simulink model "et_robocon_dev_guy_arch_pi"  (R2013b)
settings: Solver=FixedStepDiscrete  SolverMode=SingleTasking  StartTime=0.0  StopTime=inf  FixedStep=balancer_ts  RelTol=1e-3
undefined symbols (not defined in the file): a_d, a_r, balancerStates_Bus0, Batt, battery_gain, battery_offset, cmd_max, current_mode_status, current_task_operation_status, DiscIntNeverNeededParam, exec_period, Init_Bus0, K, k_f, k_i, k_phidot, k_thetadot, lightCalib, R, STATE, TRACK_MODE_LIST, ts2, W
libraries: legonxtlib x28, simulink x19, simulink_extras x4
(part 3 of 4)

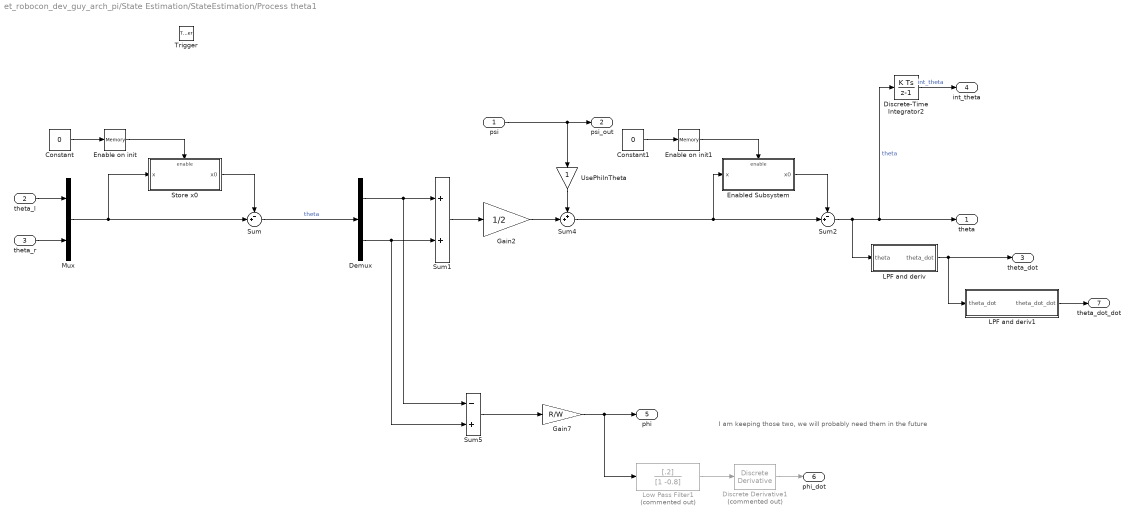
== system et_robocon_dev_guy_arch_pi/State Estimation/StateEstimation/Process theta1 ==
  note: I am keeping those two, we will probably need them in the future
  psi : Inport
  theta_l : Inport  Port=2
  theta_r : Inport  Port=3
  Trigger : TriggerPort  TriggerType=function-call  StatesWhenEnabling=reset  PortDimensions=1
  Constant : Constant  Value=0  OutDataTypeStr=boolean
  Constant1 : Constant  Value=0  OutDataTypeStr=boolean
  Demux : Demux  Outputs=2
  Discrete Derivative1 : simulink/Discrete/Discrete Derivative  Commented=on  gainval=1.0  ICPrevScaledInput=0.0  InputProcessing=Inherited  OutMin=[]  OutMax=[]  OutDataType=fixdt(1, 16)  OutScaling=2^-10  DoSatur=off
  Discrete-Time Integrator2 : DiscreteIntegrator  SampleTime=-1  ICPrevOutput=DiscIntNeverNeededParam  ICPrevScaledInput=DiscIntNeverNeededParam
  Enable on init : Memory  X0=1  InheritSampleTime=on
  Enable on init1 : Memory  X0=1  InheritSampleTime=on
  Enabled Subsystem : Subsystem  TreatAsAtomicUnit=on
  Gain2 : Gain  Gain=1/2
  Gain7 : Gain  Gain=R/W
  LPF and deriv : Subsystem
  LPF and deriv1 : Subsystem
  Low Pass Filter1 : DiscreteFilter  Commented=on  Numerator=[.2]  Denominator=[1 -0.8]
  Mux : Mux  Inputs=2
  Store x0 : Subsystem  TreatAsAtomicUnit=on
  Sum : Sum  Inputs=-+|
  Sum1 : Sum
  Sum2 : Sum  Inputs=-+|
  Sum4 : Sum  Inputs=++|
  Sum5 : Sum  Inputs=-+
  UsePhiInTheta : Gain
  theta : Outport  InitialOutput=0
  psi_out : Outport  Port=2  InitialOutput=0
  theta_dot : Outport  Port=3  OutputWhenDisabled=reset  InitialOutput=0
  int_theta : Outport  Port=4  InitialOutput=0
  phi : Outport  Port=5  OutputWhenDisabled=reset  InitialOutput=0
  phi_dot : Outport  Port=6  OutputWhenDisabled=reset  InitialOutput=0
  theta_dot_dot : Outport  Port=7  OutputWhenDisabled=reset  InitialOutput=0
  wires:
  Gain7/1 -> Low Pass Filter1/1, phi/1
  Sum5/1 -> Gain7/1
  Sum2/1 -> LPF and deriv/1(theta), theta/1, Discrete-Time Integrator2/1  "theta"
  Enabled Subsystem/1(x0) -> Sum2/1
  Constant1/1 -> Enable on init1/1
  Enable on init1/1 -> Enabled Subsystem/Enable
  Sum4/1 -> Sum2/2, Enabled Subsystem/1(x)
  Discrete-Time Integrator2/1 -> int_theta/1  "int_theta"
  psi/1 -> UsePhiInTheta/1, psi_out/1
  UsePhiInTheta/1 -> Sum4/1
  Sum1/1 -> Gain2/1
  Gain2/1 -> Sum4/2
  Demux/2 -> Sum1/2, Sum5/2
  Demux/1 -> Sum1/1, Sum5/1
  theta_r/1 -> Mux/2
  theta_l/1 -> Mux/1
  Mux/1 -> Sum/2, Store x0/1(x)
  Sum/1 -> Demux/1  "theta"
  Store x0/1(x0) -> Sum/1
  Constant/1 -> Enable on init/1
  Enable on init/1 -> Store x0/Enable
  Low Pass Filter1/1 -> Discrete Derivative1/1
  Discrete Derivative1/1 -> phi_dot/1
  LPF and deriv/1(theta_dot) -> LPF and deriv1/1(theta_dot), theta_dot/1
  LPF and deriv1/1(theta_dot_dot) -> theta_dot_dot/1

== system et_robocon_dev_guy_arch_pi/Main Controller/normal_operation_modes.line_tracking_after_seesaw/line_tracking_mode.Track.analyzeEncoders/AngleCounter/AngleCount_and_EncoderReset ==
  In1 : Inport
  In2 : Inport  Port=2  OutDataTypeStr=uint8
  Trigger : TriggerPort
  Data Store Read : DataStoreRead  Commented=on  DataStoreName=fwd_premode_last
  Data Store Write : DataStoreWrite  Commented=on  DataStoreName=fwd_postmode_init
  EC : Outport
  Cnt : Outport  Port=2  InitialOutput=1
  wires:
  In2/1 -> Cnt/1
  In1/1 -> EC/1
  Data Store Read/1 -> Data Store Write/1

== system et_robocon_dev_guy_arch_pi/Main Controller/normal_operation_modes.line_tracking_after_seesaw/line_tracking_mode.Track.analyzeEncoders/AngleCounter/Compute Distance ==
  R : Inport
  L : Inport  Port=2
  Gain1 : Gain  Gain=1/2
  Subtract : Sum
  EncoderMean : Outport
  wires:
  Gain1/1 -> EncoderMean/1
  Subtract/1 -> Gain1/1
  L/1 -> Subtract/2
  R/1 -> Subtract/1

== system et_robocon_dev_guy_arch_pi/Main Controller/normal_operation_modes.line_tracking_after_seesaw/line_tracking_mode.Track.analyzeEncoders/AngleCounter/Direction ==
  note: 160: Distance between left tire and right tire
      | 41: Radius of tire
  R : Inport
  L : Inport  Port=2
  Gain2 : Gain  Gain=41/160
  Subtract1 : Sum  Inputs=+-
  Angle : Outport
  wires:
  Gain2/1 -> Angle/1
  R/1 -> Subtract1/1
  L/1 -> Subtract1/2
  Subtract1/1 -> Gain2/1

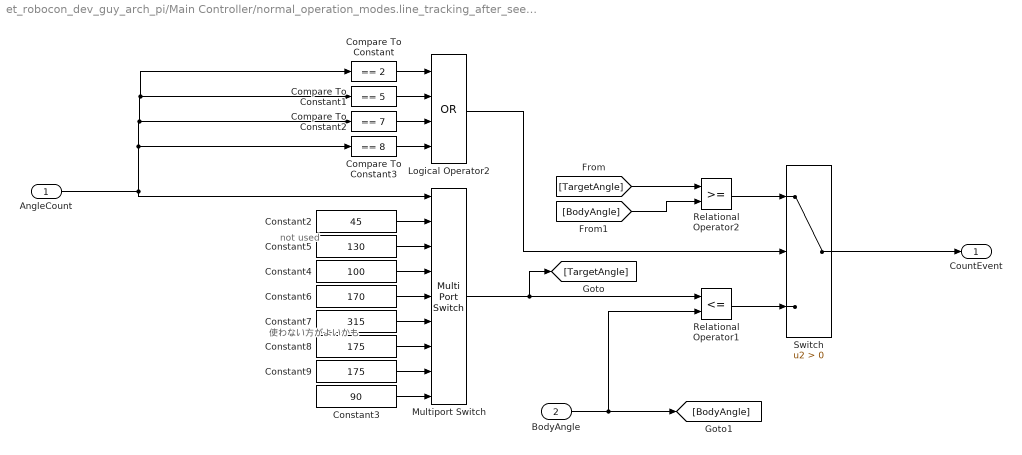
== system et_robocon_dev_guy_arch_pi/Main Controller/normal_operation_modes.line_tracking_after_seesaw/line_tracking_mode.Track.analyzeEncoders/AngleCounter/JudgeByAngle ==
  note: not used
  note: 使わない方がよいかも
  AngleCount : Inport
  BodyAngle : Inport  Port=2
  Compare To Constant : simulink/Logic and Bit Operations/Compare To Constant  relop===  const=2  OutDataTypeStr=boolean
  Compare To Constant1 : simulink/Logic and Bit Operations/Compare To Constant  relop===  const=5  OutDataTypeStr=boolean
  Compare To Constant2 : simulink/Logic and Bit Operations/Compare To Constant  relop===  const=7  OutDataTypeStr=boolean
  Compare To Constant3 : simulink/Logic and Bit Operations/Compare To Constant  relop===  const=8  OutDataTypeStr=boolean
  Constant2 : Constant  Value=45  OutDataTypeStr=int32
  Constant3 : Constant  Value=90  OutDataTypeStr=int32
  Constant4 : Constant  Value=100  OutDataTypeStr=int32
  Constant5 : Constant  Value=130  OutDataTypeStr=int32
  Constant6 : Constant  Value=170  OutDataTypeStr=int32
  Constant7 : Constant  Value=315  OutDataTypeStr=int32
  Constant8 : Constant  Value=175  OutDataTypeStr=int32
  Constant9 : Constant  Value=175  OutDataTypeStr=int32
  Logical Operator2 : Logic  Operator=OR  Inputs=4  AllPortsSameDT=off  OutDataTypeStr=boolean
  Multiport Switch : MultiPortSwitch  Inputs=8  DiagnosticForDefault=None
  Relational Operator1 : RelationalOperator  Operator=<=  OutDataTypeStr=boolean
  Relational Operator2 : RelationalOperator  OutDataTypeStr=boolean
  Switch : Switch  Criteria=u2 > Threshold
  CountEvent : Outport
  wires:
  Constant3/1 -> Multiport Switch/9
  Relational Operator1/1 -> Switch/3
  Compare To Constant2/1 -> Logical Operator2/3
  Compare To Constant3/1 -> Logical Operator2/4
  Compare To Constant1/1 -> Logical Operator2/2
  Compare To Constant/1 -> Logical Operator2/1
  Relational Operator2/1 -> Switch/1
  Logical Operator2/1 -> Switch/2
  AngleCount/1 -> Compare To Constant/1, Compare To Constant1/1, Compare To Constant2/1, Compare To Constant3/1, Multiport Switch/1
  BodyAngle/1 -> [BodyAngle], Relational Operator1/2
  Constant9/1 -> Multiport Switch/8
  Multiport Switch/1 -> [TargetAngle], Relational Operator1/1
  Constant4/1 -> Multiport Switch/4
  Constant8/1 -> Multiport Switch/7
  Constant5/1 -> Multiport Switch/3
  Constant2/1 -> Multiport Switch/2
  Constant6/1 -> Multiport Switch/5
  Constant7/1 -> Multiport Switch/6
  [BodyAngle] -> Relational Operator2/2
  [TargetAngle] -> Relational Operator2/1
  Switch/1 -> CountEvent/1

== system et_robocon_dev_guy_arch_pi/Main Controller/normal_operation_modes.line_tracking_after_seesaw/line_tracking_mode.Track.analyzeEncoders/AngleCounter/JudgeByDistance ==
  AngleCount : Inport
  Distance : Inport  Port=2
  Constant1 : Constant  Value=14700  OutDataTypeStr=int32
  Constant10 : Constant  Value=9700  OutDataTypeStr=int32
  Constant2 : Constant  Value=6220  OutDataTypeStr=int32
  Constant3 : Constant  Value=18700  OutDataTypeStr=int32
  Constant4 : Constant  Value=11550  OutDataTypeStr=int32
  Constant5 : Constant  Value=8000  OutDataTypeStr=int32
  Constant6 : Constant  Value=12000  OutDataTypeStr=int32
  Constant7 : Constant  Value=11800  OutDataTypeStr=int32
  Constant8 : Constant  Value=17100  OutDataTypeStr=int32
  Constant9 : Constant  Value=17800  OutDataTypeStr=int32
  Multiport Switch : MultiPortSwitch  Inputs=8  DiagnosticForDefault=None
  Relational Operator2 : RelationalOperator  Operator=<=  OutDataTypeStr=boolean
  StartDistance : Constant  Value=0  OutDataTypeStr=int32
  Sum2 : Sum  Inputs=|+-
  Terminator : Terminator
  Terminator1 : Terminator
  CountEvent : Outport
  wires:
  Constant1/1 -> Multiport Switch/6
  Constant6/1 -> Multiport Switch/5
  Constant2/1 -> Multiport Switch/2
  Constant5/1 -> Multiport Switch/3
  Constant8/1 -> Multiport Switch/7
  Constant4/1 -> Multiport Switch/4
  Constant9/1 -> Multiport Switch/8
  Distance/1 -> Relational Operator2/2
  Constant3/1 -> Multiport Switch/9
  Multiport Switch/1 -> Sum2/1
  StartDistance/1 -> Sum2/2
  Sum2/1 -> Relational Operator2/1
  Relational Operator2/1 -> CountEvent/1
  AngleCount/1 -> Multiport Switch/1
  Constant7/1 -> Terminator/1
  Constant10/1 -> Terminator1/1

== system et_robocon_dev_guy_arch_pi/Main Controller/normal_operation_modes.line_tracking_after_seesaw/line_tracking_mode.Track.lineTracker/Handler/rocket_start ==
  fwd : Inport
  Constant : Constant  Value=2  OutDataTypeStr=single  SampleTime=-1
  Saturation : Saturate  UpperLimit=200  LowerLimit=0  RndMeth=Simplest
  Sum : Sum  Inputs=|++  AccumDataTypeStr=single  OutDataTypeStr=single  RndMeth=Simplest  InputSameDT=on
  Sum1 : Sum  Inputs=-+  AccumDataTypeStr=single  OutDataTypeStr=single  RndMeth=Simplest
  Switch : Switch  Criteria=u2 > Threshold  OutDataTypeStr=single  RndMeth=Simplest
  Unit Delay1 : UnitDelay  InitialCondition=100  SampleTime=-1
  fwd_slow : Outport
  wires:
  Saturation/1 -> Switch/3, Sum1/2
  fwd/1 -> Switch/1, Sum1/1
  Switch/1 -> fwd_slow/1
  Sum1/1 -> Switch/2
  Sum/1 -> Saturation/1, Unit Delay1/1
  Constant/1 -> Sum/1
  Unit Delay1/1 -> Sum/2

== system et_robocon_dev_guy_arch_pi/Main Controller/normal_operation_modes.line_tracking_after_seesaw/line_tracking_mode.Track.lineTracker/Handler/slow_start ==
  fwd : Inport
  Constant : Constant  Value=2  OutDataTypeStr=single  SampleTime=-1
  Saturation : Saturate  UpperLimit=200  LowerLimit=0  RndMeth=Simplest
  Sum : Sum  Inputs=|++  AccumDataTypeStr=single  OutDataTypeStr=single  RndMeth=Simplest  InputSameDT=on
  Sum1 : Sum  Inputs=-+  AccumDataTypeStr=single  OutDataTypeStr=single  RndMeth=Simplest
  Switch : Switch  Criteria=u2 > Threshold  OutDataTypeStr=single  RndMeth=Simplest
  Unit Delay1 : UnitDelay  InitialCondition=30  SampleTime=-1
  fwd_slow : Outport
  wires:
  Saturation/1 -> Switch/3, Sum1/2
  fwd/1 -> Switch/1, Sum1/1
  Switch/1 -> fwd_slow/1
  Sum1/1 -> Switch/2
  Sum/1 -> Saturation/1, Unit Delay1/1
  Constant/1 -> Sum/1
  Unit Delay1/1 -> Sum/2

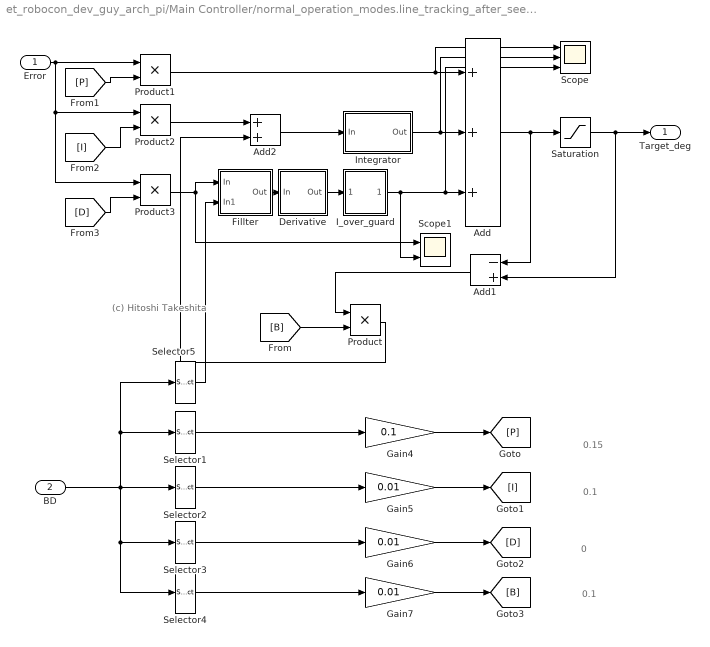
== system et_robocon_dev_guy_arch_pi/Main Controller/normal_operation_modes.line_tracking_after_seesaw/line_tracking_mode.Track.lineTracker/SwitchForFreeSteering/tmpController ==
  note: (c) Hitoshi Takeshita
  note: 0.15
  note: 0.1
  note: 0
  note: 0.1
  Error : Inport
  BD : Inport  Port=2
  Add : Sum  Inputs=+++  OutDataTypeStr=single  RndMeth=Nearest
  Add1 : Sum  Inputs=-+  OutDataTypeStr=single  RndMeth=Nearest
  Add2 : Sum  OutDataTypeStr=single  RndMeth=Nearest
  Derivative : Subsystem  mask{Ts_=Ts_}
      mask prompts: Ts_ "Sampling Time"
      mask init:
      | Ts_=Ts_;
      mask Display: dpoly([1 -1],[0 Ts_],'z')
  Fillter : Subsystem
  Gain4 : Gain  Gain=0.1
  Gain5 : Gain  Gain=0.01
  Gain6 : Gain  Gain=0.01
  Gain7 : Gain  Gain=0.01
  I_over_guard : Subsystem
  Integrator : Subsystem  mask{Ts_=Ts_}
      mask prompts: Ts_ "Sampling Time"
      mask Display: dpoly([Ts_],[1 -1],'z')
  Product{,1..3} (4 alike) : Product  RndMeth=Zero
  Saturation : Saturate  UpperLimit=SaturationMax  LowerLimit=SaturationMin  LinearizeAsGain=off  OutDataTypeStr=single  RndMeth=Nearest
  Scope : Scope  NumInputPorts=3
      settings: YMin=-5~-5~-5  YMax=5~5~5  SaveName=ScopeData5
  Scope1 : Scope  NumInputPorts=2
      settings: YMin=-5~-5  YMax=5~5  SaveName=ScopeData6
  Selector1 : Selector  InputPortWidth=5  IndexOptions=Index vector (dialog)  Indices=1  OutputSizes=1
  Selector2 : Selector  InputPortWidth=5  IndexOptions=Index vector (dialog)  Indices=2  OutputSizes=1
  Selector3 : Selector  InputPortWidth=5  IndexOptions=Index vector (dialog)  Indices=3  OutputSizes=1
  Selector4 : Selector  InputPortWidth=5  IndexOptions=Index vector (dialog)  Indices=4  OutputSizes=1
  Selector5 : Selector  InputPortWidth=5  IndexOptions=Index vector (dialog)  Indices=5  OutputSizes=1
  Target_deg : Outport
  wires:
  Product/1 -> Add2/2
  Add1/1 -> Product/1
  Add2/1 -> Integrator/1(In)
  Product1/1 -> Add/1, Scope/1
  Integrator/1(Out) -> Add/2, Scope/2
  Add/1 -> Add1/1, Saturation/1
  Derivative/1(Out) -> I_over_guard/1(In1)
  Product2/1 -> Add2/1
  Product3/1 -> Scope1/1, Fillter/1(In)
  Saturation/1 -> Add1/2, Target_deg/1
  Selector1/1 -> Gain4/1
  Selector2/1 -> Gain5/1
  Selector3/1 -> Gain6/1
  Selector4/1 -> Gain7/1
  Gain4/1 -> [P]
  Gain5/1 -> [I]
  Gain6/1 -> [D]
  Gain7/1 -> [B]
  [B] -> Product/2
  [P] -> Product1/2
  [I] -> Product2/2
  [D] -> Product3/2
  BD/1 -> Selector2/1, Selector3/1, Selector4/1, Selector1/1, Selector5/1
  Error/1 -> Product1/1, Product2/1, Product3/1
  I_over_guard/1(Out1) -> Add/3, Scope/3, Scope1/2
  Fillter/1(Out) -> Derivative/1(In)
  Selector5/1 -> Fillter/2(In1)

== system et_robocon_dev_guy_arch_pi/Main Controller/normal_operation_modes.line_tracking_after_seesaw/line_tracking_mode.balanceControl/ForSimulation/Cal_PWM ==
  note: Calculate maximum of DC motor
      | voltatege from battery using an
      | experimental expression.
  note: Turn NXTway-GS by applying pwm offset
      | to left and right motor in the counter direction.
  pwm_turn : Inport
  err : Inport  Port=2
  battery : Inport  Port=3
  Cal_vol_max : Subsystem
  Gain : Gain  Gain=100  OutDataTypeStr=Inherit: Same as input  ParamDataTypeStr=Inherit: Same as input
  Product : Product  Inputs=*/  RndMeth=Simplest  OutDataTypeStr=Inherit: Same as first input
  Sum : Sum  Inputs=|++  OutDataTypeStr=Inherit: Same as first input
  Sum1 : Sum  Inputs=|+-  OutDataTypeStr=Inherit: Same as first input
  pwm_l_limiter : Saturate  UpperLimit=100  LowerLimit=-100
      settings: AttributesFormatString=max = %<UpperLimit>\nmin = %<LowerLimit>
  pwm_r_limiter : Saturate  UpperLimit=100  LowerLimit=-100
      settings: AttributesFormatString=max = %<UpperLimit>\nmin = %<LowerLimit>
  pwm_l : Outport
  pwm_r : Outport  Port=2
  wires:
  Sum/1 -> pwm_l_limiter/1
  pwm_turn/1 -> Sum/2, Sum1/2
  Gain/1 -> Sum1/1, Sum/1
  err/1 -> Product/1
  Product/1 -> Gain/1
  battery/1 -> Cal_vol_max/1(battery)
  Cal_vol_max/1(vol_max) -> Product/2
  Sum1/1 -> pwm_r_limiter/1
  pwm_r_limiter/1 -> pwm_r/1
  pwm_l_limiter/1 -> pwm_l/1

== system et_robocon_dev_guy_arch_pi/Main Controller/normal_operation_modes.line_tracking_after_seesaw/line_tracking_mode.balanceControl/ForSimulation/Cal_Reference ==
  note: Divide command values by
      | maximum of command input.
  note: Smooth velocity command
      | using Low Path Filter to
      | suppress rapid input change.
  cmd_forward : Inport
  cmd_turn : Inport  Port=2
  Constant1 : Constant  Value=cmd_max  VectorParams1D=off  OutDataTypeStr=single  SampleTime=-1
      settings: AttributesFormatString=DataType = %<OutDataTypeStr>
  Constant2 : Constant  Value=0  VectorParams1D=off  OutDataTypeStr=single  SampleTime=-1
      settings: AttributesFormatString=DataType = %<OutDataTypeStr>
  Constant3 : Constant  Value=0  VectorParams1D=off  OutDataTypeStr=single  SampleTime=-1
      settings: AttributesFormatString=DataType = %<OutDataTypeStr>
  Constant6 : Constant  Value=cmd_max  VectorParams1D=off  OutDataTypeStr=single  SampleTime=-1
      settings: AttributesFormatString=DataType = %<OutDataTypeStr>
  DiscreteIntegrator : Subsystem
  Divide : Product  Inputs=*/  RndMeth=Simplest  OutDataTypeStr=Inherit: Same as first input
  Divide1 : Product  Inputs=*/  RndMeth=Simplest  OutDataTypeStr=Inherit: Same as first input
  Gain1 : Gain  Gain=k_thetadot  OutDataTypeStr=Inherit: Same as input  ParamDataTypeStr=Inherit: Same as input
  Gain2 : Gain  Gain=k_phidot  OutDataTypeStr=Inherit: Same as input  ParamDataTypeStr=Inherit: Same as input
  LowPathFilter : Subsystem
  Mux : Mux
  pwm_turn : Outport
  theta_ref : Outport  Port=2
  x1_ref : Outport  Port=3
  wires:
  cmd_turn/1 -> Divide1/1
  Gain1/1 -> LowPathFilter/1(in)
  cmd_forward/1 -> Divide/1
  Divide/1 -> Gain1/1
  Gain2/1 -> pwm_turn/1  "pwm_turn"
  Constant1/1 -> Divide1/2
  Divide1/1 -> Gain2/1
  Mux/1 -> x1_ref/1
  DiscreteIntegrator/1(out) -> theta_ref/1, Mux/1  "theta_ref"
  Constant2/1 -> Mux/2  "psi_ref"
  Constant3/1 -> Mux/4  "psidot_ref"
  LowPathFilter/1(out) -> Mux/3, DiscreteIntegrator/1(in)  "thetadot_ref"
  Constant6/1 -> Divide/2

== system et_robocon_dev_guy_arch_pi/Main Controller/normal_operation_modes.line_tracking_after_seesaw/line_tracking_mode.balanceControl/ForSimulation/Cal_x1 ==
  note: Smooth measured velocity value using
      | Low Path Filter to reduce the noise
      | because it makes extra control input.
  note: Calculate gyro offset for removing gyro drift.
  gyro : Inport
  gyro_offset : Inport  Port=2
  theta_m_l : Inport  Port=3
  theta_m_r : Inport  Port=4
  DiscreteDerivative : Subsystem
  DiscreteIntegrator : Subsystem
  Gain : Gain  Gain=1/2  OutDataTypeStr=Inherit: Same as input  ParamDataTypeStr=Inherit: Same as input
  LowPathFilter : Subsystem
  Mux1 : Mux
  Sum1 : Sum  Inputs=++|  OutDataTypeStr=Inherit: Same as first input
  Sum2 : Sum  Inputs=|+-  OutDataTypeStr=Inherit: Same as first input
  Sum4 : Sum  Inputs=|++  OutDataTypeStr=Inherit: Same as first input
  Sum6 : Sum  Inputs=|++  OutDataTypeStr=Inherit: Same as first input
  deg2rad : Gain  Gain=deg2rad  OutDataTypeStr=Inherit: Same as input  ParamDataTypeStr=Inherit: Same as input
  deg2rad1 : Gain  Gain=deg2rad  OutDataTypeStr=Inherit: Same as input  ParamDataTypeStr=Inherit: Same as input
  deg2rad2 : Gain  Gain=deg2rad  OutDataTypeStr=Inherit: Same as input  ParamDataTypeStr=Inherit: Same as input
  theta : Outport
  x1 : Outport  Port=2
  wires:
  deg2rad1/1 -> Sum4/1
  Mux1/1 -> x1/1
  DiscreteIntegrator/1(out) -> Sum6/2, Sum4/2, Mux1/2  "psi"
  deg2rad/1 -> Sum6/1
  theta_m_l/1 -> deg2rad/1
  theta_m_r/1 -> deg2rad1/1
  DiscreteDerivative/1(out) -> Mux1/3  "thetadot"
  Sum6/1 -> Sum1/1  "theta_l"
  Sum4/1 -> Sum1/2  "theta_r"
  Sum1/1 -> Gain/1  "thata_m_sum"
  gyro/1 -> Sum2/1
  Sum2/1 -> deg2rad2/1
  deg2rad2/1 -> Mux1/4, DiscreteIntegrator/1(in)  "psidot"
  LowPathFilter/1(out) -> DiscreteDerivative/1(in)
  Gain/1 -> theta/1, Mux1/1, LowPathFilter/1(in)  "theta"
  gyro_offset/1 -> Sum2/2
  LowPathFilter/2(out1) -> DiscreteDerivative/2(in1)

== system et_robocon_dev_guy_arch_pi/Main Controller/normal_operation_modes.line_tracking_after_seesaw/line_tracking_mode.balanceControl/ForSimulation/DiscreteIntegrator ==
  in : Inport
  Gain : Gain  Gain=exec_period  OutDataTypeStr=Inherit: Same as input  ParamDataTypeStr=Inherit: Same as input
  Sum : Sum  Inputs=|++  OutDataTypeStr=Inherit: Same as first input
  Unit Delay : UnitDelay  SampleTime=-1  StateName=ud_psi  StateMustResolveToSignalObject=on
      settings: AttributesFormatString=Signal name = ud_psi
  out : Outport
  wires:
  Unit Delay/1 -> Sum/2, out/1
  Gain/1 -> Sum/1
  Sum/1 -> Unit Delay/1
  in/1 -> Gain/1

== system et_robocon_dev_guy_arch_pi/Main Controller/normal_operation_modes.line_tracking_after_seesaw/line_tracking_mode.balanceControl/Low Pass Filter/Store Offset ==
  x : Inport
  Enable : EnablePort
  x0 : Outport  InitialOutput=0
  wires:
  x/1 -> x0/1

== system et_robocon_dev_guy_arch_pi/Main Controller/normal_operation_modes.line_tracking_after_seesaw/line_tracking_mode.balanceControl/removeOffset/Store x0 ==
  In1 : Inport
  In2 : Inport  Port=2
  Enable : EnablePort
  Out1 : Outport
  Out2 : Outport  Port=2
  wires:
  In1/1 -> Out1/1
  In2/1 -> Out2/1

== system et_robocon_dev_guy_arch_pi/Main Controller/normal_operation_modes.line_tracking_mode/line_tracking_mode.Track.analyzeEncoders/AngleCounter/AngleCount_and_EncoderReset ==
  In1 : Inport
  In2 : Inport  Port=2  OutDataTypeStr=uint8
  Trigger : TriggerPort
  Data Store Read : DataStoreRead  Commented=on  DataStoreName=fwd_premode_last
  Data Store Write : DataStoreWrite  Commented=on  DataStoreName=fwd_postmode_init
  EC : Outport
  Cnt : Outport  Port=2  InitialOutput=1
  wires:
  In2/1 -> Cnt/1
  In1/1 -> EC/1
  Data Store Read/1 -> Data Store Write/1

== system et_robocon_dev_guy_arch_pi/Main Controller/normal_operation_modes.line_tracking_mode/line_tracking_mode.Track.analyzeEncoders/AngleCounter/Compute Distance ==
  R : Inport
  L : Inport  Port=2
  Gain1 : Gain  Gain=1/2
  Subtract : Sum
  EncoderMean : Outport
  wires:
  Gain1/1 -> EncoderMean/1
  Subtract/1 -> Gain1/1
  L/1 -> Subtract/2
  R/1 -> Subtract/1

== system et_robocon_dev_guy_arch_pi/Main Controller/normal_operation_modes.line_tracking_mode/line_tracking_mode.Track.analyzeEncoders/AngleCounter/Direction ==
  note: 160: Distance between left tire and right tire
      | 41: Radius of tire
  R : Inport
  L : Inport  Port=2
  Gain2 : Gain  Gain=41/160
  Subtract1 : Sum  Inputs=+-
  Angle : Outport
  wires:
  Gain2/1 -> Angle/1
  R/1 -> Subtract1/1
  L/1 -> Subtract1/2
  Subtract1/1 -> Gain2/1

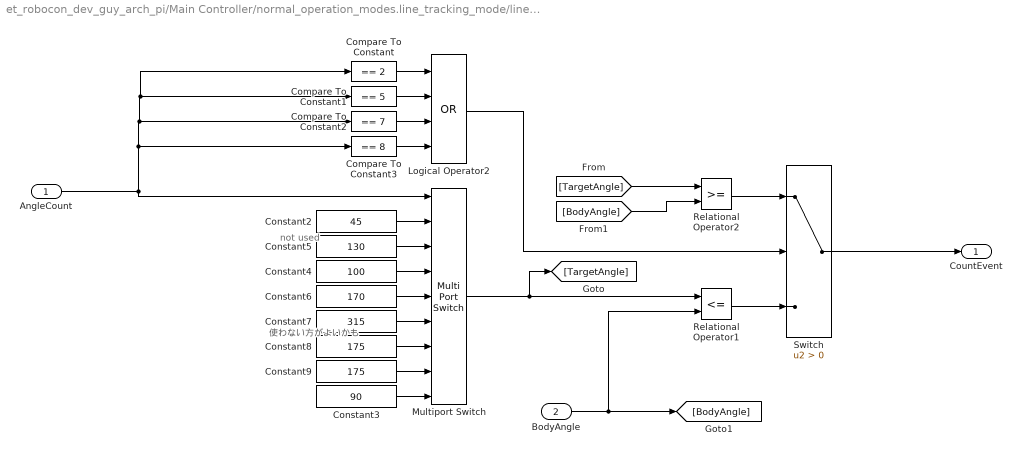
== system et_robocon_dev_guy_arch_pi/Main Controller/normal_operation_modes.line_tracking_mode/line_tracking_mode.Track.analyzeEncoders/AngleCounter/JudgeByAngle ==
  note: not used
  note: 使わない方がよいかも
  AngleCount : Inport
  BodyAngle : Inport  Port=2
  Compare To Constant : simulink/Logic and Bit Operations/Compare To Constant  relop===  const=2  OutDataTypeStr=boolean
  Compare To Constant1 : simulink/Logic and Bit Operations/Compare To Constant  relop===  const=5  OutDataTypeStr=boolean
  Compare To Constant2 : simulink/Logic and Bit Operations/Compare To Constant  relop===  const=7  OutDataTypeStr=boolean
  Compare To Constant3 : simulink/Logic and Bit Operations/Compare To Constant  relop===  const=8  OutDataTypeStr=boolean
  Constant2 : Constant  Value=45  OutDataTypeStr=int32
  Constant3 : Constant  Value=90  OutDataTypeStr=int32
  Constant4 : Constant  Value=100  OutDataTypeStr=int32
  Constant5 : Constant  Value=130  OutDataTypeStr=int32
  Constant6 : Constant  Value=170  OutDataTypeStr=int32
  Constant7 : Constant  Value=315  OutDataTypeStr=int32
  Constant8 : Constant  Value=175  OutDataTypeStr=int32
  Constant9 : Constant  Value=175  OutDataTypeStr=int32
  Logical Operator2 : Logic  Operator=OR  Inputs=4  AllPortsSameDT=off  OutDataTypeStr=boolean
  Multiport Switch : MultiPortSwitch  Inputs=8  DiagnosticForDefault=None
  Relational Operator1 : RelationalOperator  Operator=<=  OutDataTypeStr=boolean
  Relational Operator2 : RelationalOperator  OutDataTypeStr=boolean
  Switch : Switch  Criteria=u2 > Threshold
  CountEvent : Outport
  wires:
  Constant3/1 -> Multiport Switch/9
  Relational Operator1/1 -> Switch/3
  Compare To Constant2/1 -> Logical Operator2/3
  Compare To Constant3/1 -> Logical Operator2/4
  Compare To Constant1/1 -> Logical Operator2/2
  Compare To Constant/1 -> Logical Operator2/1
  Relational Operator2/1 -> Switch/1
  Logical Operator2/1 -> Switch/2
  AngleCount/1 -> Compare To Constant/1, Compare To Constant1/1, Compare To Constant2/1, Compare To Constant3/1, Multiport Switch/1
  BodyAngle/1 -> [BodyAngle], Relational Operator1/2
  Constant9/1 -> Multiport Switch/8
  Multiport Switch/1 -> [TargetAngle], Relational Operator1/1
  Constant4/1 -> Multiport Switch/4
  Constant8/1 -> Multiport Switch/7
  Constant5/1 -> Multiport Switch/3
  Constant2/1 -> Multiport Switch/2
  Constant6/1 -> Multiport Switch/5
  Constant7/1 -> Multiport Switch/6
  [BodyAngle] -> Relational Operator2/2
  [TargetAngle] -> Relational Operator2/1
  Switch/1 -> CountEvent/1

== system et_robocon_dev_guy_arch_pi/Main Controller/normal_operation_modes.line_tracking_mode/line_tracking_mode.Track.analyzeEncoders/AngleCounter/JudgeByDistance ==
  AngleCount : Inport
  Distance : Inport  Port=2
  Constant1 : Constant  Value=14700  OutDataTypeStr=int32
  Constant10 : Constant  Value=9700  OutDataTypeStr=int32
  Constant2 : Constant  Value=6220  OutDataTypeStr=int32
  Constant3 : Constant  Value=18700  OutDataTypeStr=int32
  Constant4 : Constant  Value=11550  OutDataTypeStr=int32
  Constant5 : Constant  Value=8000  OutDataTypeStr=int32
  Constant6 : Constant  Value=12000  OutDataTypeStr=int32
  Constant7 : Constant  Value=11800  OutDataTypeStr=int32
  Constant8 : Constant  Value=17100  OutDataTypeStr=int32
  Constant9 : Constant  Value=17800  OutDataTypeStr=int32
  Multiport Switch : MultiPortSwitch  Inputs=8  DiagnosticForDefault=None
  Relational Operator2 : RelationalOperator  Operator=<=  OutDataTypeStr=boolean
  StartDistance : Constant  Value=0  OutDataTypeStr=int32
  Sum2 : Sum  Inputs=|+-
  Terminator : Terminator
  Terminator1 : Terminator
  CountEvent : Outport
  wires:
  Constant1/1 -> Multiport Switch/6
  Constant6/1 -> Multiport Switch/5
  Constant2/1 -> Multiport Switch/2
  Constant5/1 -> Multiport Switch/3
  Constant8/1 -> Multiport Switch/7
  Constant4/1 -> Multiport Switch/4
  Constant9/1 -> Multiport Switch/8
  Distance/1 -> Relational Operator2/2
  Constant3/1 -> Multiport Switch/9
  Multiport Switch/1 -> Sum2/1
  StartDistance/1 -> Sum2/2
  Sum2/1 -> Relational Operator2/1
  Relational Operator2/1 -> CountEvent/1
  AngleCount/1 -> Multiport Switch/1
  Constant7/1 -> Terminator/1
  Constant10/1 -> Terminator1/1

== stateflow chart et_robocon_dev_guy_arch_pi/Main Controller/normal_operation_modes.line_tracking_after_seesaw ==
  state line_tracking_mode
    entry:
    desired_tail = single(0); %radian
    entry, during:
    PWM.tail = tail_controller(sensors.theta_T,desired_tail);
    exit:
    PWM.tail = single(0);
    state ResetStates
      entry:
      initFlags.theta = single(1);
      initFlags.gyroReset = single(1);
    state ResetDone
      entry:
      initFlags.theta = single(0);
      initFlags.gyroReset = single(0);
    state Track
      entry:
      debugFlag = uint16(401);
      bias = single(0);
      FlagSteering = single(0);
      minLight = single(-75);
      maxLight = single(67);
      lineSide = single(1);
      enablePhiTracking = single(0);
      state preProcess [parallel]
        during:
        on every(3, tick):
        [normalizedLight, filteredLight] = processLight(sensors.light, bias, minLight,maxLight);
        [AngleCount,EncoderReset,Angle, Distance] = analyzeEncoders(rawSensors);
        settings: executionOrder=1
      state manageRacePhases [parallel]
        settings: executionOrder=2
        state ApproahSeesawtransition3
          entry:
          Speak;
          PID = single([0 0 0 0 0]');
          bias = single(0);
          FlagSteering = single(1);
          lineSide = single(-1);
          phi_tmp  =single(0);
          enablePhiTracking = single(1);
          state accelerate1
            during:
            fwd = fwd + single(1/3);
          state coast1
          (default) -> line_tracking_mode.Track.manageRacePhases.ApproahSeesawtransition3.accelerate1
          line_tracking_mode.Track.manageRacePhases.ApproahSeesawtransition3.accelerate1 -> line_tracking_mode.Track.manageRacePhases.ApproahSeesawtransition3.coast1 : [fwd >= 20]
        state SlowlyRestartLineTracking
          entry: Speak;
          PID = single([30 0 25 0 100]');
          bias = single(-10);
          FlagSteering = single(0);
          enablePhiTracking = single(0);
        state Bypass
          entry:
          Speak;
          PID = single([30 0 25 0 100]');
          bias = single(-10);
          FlagSteering = single(0);
          enablePhiTracking = single(0);
          state accelerate
            during:
            fwd = fwd + single(1/3);
          state coast
          (default) -> accelerate
          accelerate -> coast : [fwd >= 80]
        state ApproahSeesawtransition2
          entry:
          Speak;
          PID = single([30 0 25 0 100]');
          bias = single(-10);
          FlagSteering = single(0);
          lineSide = single(-1);
          state accelerate1
            during:
            fwd = fwd - single(1/3);
          state coast1
          (default) -> line_tracking_mode.Track.manageRacePhases.ApproahSeesawtransition2.accelerate1
          line_tracking_mode.Track.manageRacePhases.ApproahSeesawtransition2.accelerate1 -> line_tracking_mode.Track.manageRacePhases.ApproahSeesawtransition2.coast1 : [fwd <= 0]
        (default) -> ApproahSeesawtransition3
        ApproahSeesawtransition3 -> SlowlyRestartLineTracking : [filteredLight>single(0)]
        SlowlyRestartLineTracking -> Bypass : after(1,sec)
        Bypass -> ApproahSeesawtransition2 : [Distance >= single(7*360)]
      state ApplyControl [parallel]
        during:
        on every(3, tick):  lineTrackCmd = lineTracker(normalizedLight,FlagSteering,PID,fwd)
        during:
        %lineTrackCmd(2) = lineSide*lineTrackCmd(2);
        if lineSide >0
        [PWM.left PWM.right] = balanceControl(rawSensors,lineTrackCmd);
        if enablePhiTracking
        PWM.left = PWM.left + phiController(states.phi,phi_tmp,sensors.battery);
        PWM.right = PWM.right - phiController(states.phi,phi_tmp,sensors.battery);
        end
        else
        [PWM.right PWM.left] = balanceControl(rawSensors,lineTrackCmd);
        if enablePhiTracking
        PWM.left = PWM.left + phiController(states.phi,phi_tmp,sensors.battery);
        PWM.right = PWM.right - phiController(states.phi,phi_tmp,sensors.battery);
        end
        end
        dispL5(states.balancerStates.theta_dot);
        settings: executionOrder=3
      state [normalizedLight,filteredLight] = processLight(rawLight,bias,minLight,maxLight) [function]
      state [AngleCount,EncoderReset,Angle,Distance] = analyzeEncoders(rawSensors) [function]
      state cmd = lineTracker(lightSignal,flagSteering,PID,fwd) [function]
      state dispL5(x) [function]
    state SitDown
      state Stop
        during:
        lineTrackCmd = single([0 0]');
        [PWM.left PWM.right] = balanceControl(rawSensors,lineTrackCmd);
        desired_tail = single(1.6); %radian
      state Kick
        entry:
        PWM.left = single(100)
        PWM.right = single(100);
        exit:
        PWM.left = single(0)
        PWM.right = single(0);
      state Done
        entry:
        turnLightOn;
        debugFlag = uint16(402);
        PWM.left = single(0); PWM.right = single(0);
        %current_mode_status = OperationModeStatusEnum.SUCCESSFULLY_COMPLETED;
      (default) -> Stop
      Stop -> Kick : after(0.5,sec)
      Kick -> Done : after(0.2,sec)
    state cmd = phiController(phi,desiredPhi,battery) [function]
    state [leftPWM,rightPWM]  = balanceControl(rawSensors, lineTrackCmd) [function]
    state cmd = tail_controller(current,desired) [function]
    state turnLightOn [function]
    state Speak [function]
    (default) -> ResetStates
    ResetStates -> ResetDone
    ResetDone -> Track
    ApproahSeesawtransition2 -> SitDown : after(2,sec)
  data: rawLight function_input single size=1; bias function_input single size=1; normalizedLight function_output single size=1; filteredLight function_output single size=1; minLight function_input single size=1; maxLight function_input single size=1; rawSensors function_input Bus: Sensors_Bus size=1; AngleCount function_output uint8 size=1; EncoderReset function_output single size=1; Angle function_output single size=1; Distance function_output single size=1; lightSignal function_input single size=1; flagSteering function_input single size=1; PID function_input single size=5; fwd function_input single size=1; cmd function_output; x function_input double size=1; cmd function_output; phi function_input single size=1; desiredPhi function_input single size=1; battery function_input double size=1; leftPWM function_output single size=1; rawSensors function_input Bus: Sensors_Bus size=1; rightPWM function_output; lineTrackCmd function_input single size=2; current function_input single size=1; desired function_input single size=1; cmd function_output single size=1; sensors input Bus: Sensors_Bus size=1; touch input single size=1; PWM output Bus: PWM_bus size=1; debugFlag output uint16 size=1; current_mode_status data_store_memory; desired_tail local single size=1; speed_ref local single size=1; states input Bus: States_Bus size=1; rawSensors input Bus: Sensors_Bus size=1; lineTrackCmd local single size=2; PID local single size=5; normalizedLight local single size=1; AngleCount local uint8 size=1; EncoderReset local single size=1; Angle local single size=1; bias local single size=1; fwd local single size=1; FlagSteering local single size=1; filteredLight local single; EncoderTmp local single size=1; Distance local single size=1; minLight local; maxLight local; phi_tmp local single size=1; enablePhiTracking local; d0 local; lineSide local; theta_ref local; initFlags output Bus: Init_Bus size=1

== system et_robocon_dev_guy_arch_pi/Main Controller/normal_operation_modes.line_tracking_mode/line_tracking_mode.Track.lineTracker/Handler/rocket_start ==
  fwd : Inport
  Constant : Constant  Value=2  OutDataTypeStr=single  SampleTime=-1
  Saturation : Saturate  UpperLimit=200  LowerLimit=0  RndMeth=Simplest
  Sum : Sum  Inputs=|++  AccumDataTypeStr=single  OutDataTypeStr=single  RndMeth=Simplest  InputSameDT=on
  Sum1 : Sum  Inputs=-+  AccumDataTypeStr=single  OutDataTypeStr=single  RndMeth=Simplest
  Switch : Switch  Criteria=u2 > Threshold  OutDataTypeStr=single  RndMeth=Simplest
  Unit Delay1 : UnitDelay  InitialCondition=100  SampleTime=-1
  fwd_slow : Outport
  wires:
  Saturation/1 -> Switch/3, Sum1/2
  fwd/1 -> Switch/1, Sum1/1
  Switch/1 -> fwd_slow/1
  Sum1/1 -> Switch/2
  Sum/1 -> Saturation/1, Unit Delay1/1
  Constant/1 -> Sum/1
  Unit Delay1/1 -> Sum/2

== system et_robocon_dev_guy_arch_pi/Main Controller/normal_operation_modes.line_tracking_mode/line_tracking_mode.Track.lineTracker/Handler/slow_start ==
  fwd : Inport
  Constant : Constant  Value=2  OutDataTypeStr=single  SampleTime=-1
  Saturation : Saturate  UpperLimit=200  LowerLimit=0  RndMeth=Simplest
  Sum : Sum  Inputs=|++  AccumDataTypeStr=single  OutDataTypeStr=single  RndMeth=Simplest  InputSameDT=on
  Sum1 : Sum  Inputs=-+  AccumDataTypeStr=single  OutDataTypeStr=single  RndMeth=Simplest
  Switch : Switch  Criteria=u2 > Threshold  OutDataTypeStr=single  RndMeth=Simplest
  Unit Delay1 : UnitDelay  InitialCondition=30  SampleTime=-1
  fwd_slow : Outport
  wires:
  Saturation/1 -> Switch/3, Sum1/2
  fwd/1 -> Switch/1, Sum1/1
  Switch/1 -> fwd_slow/1
  Sum1/1 -> Switch/2
  Sum/1 -> Saturation/1, Unit Delay1/1
  Constant/1 -> Sum/1
  Unit Delay1/1 -> Sum/2

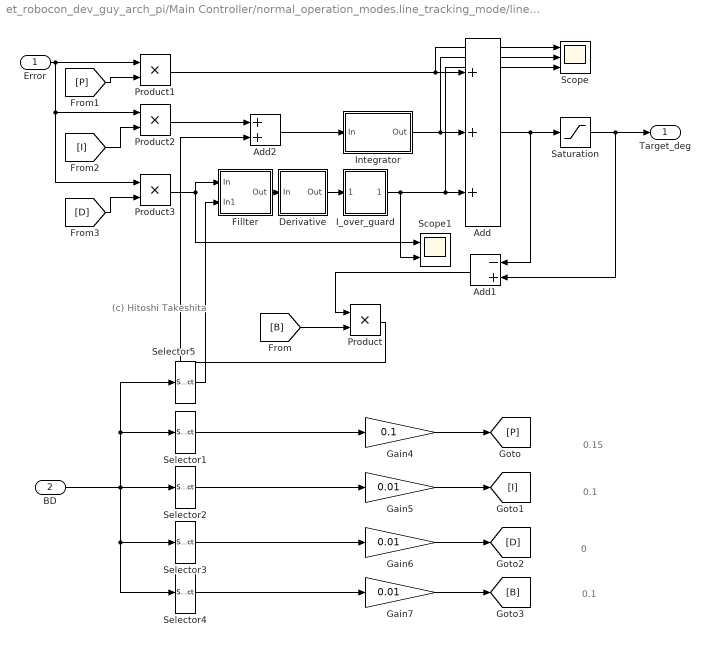
== system et_robocon_dev_guy_arch_pi/Main Controller/normal_operation_modes.line_tracking_mode/line_tracking_mode.Track.lineTracker/SwitchForFreeSteering/tmpController ==
  note: (c) Hitoshi Takeshita
  note: 0.15
  note: 0.1
  note: 0
  note: 0.1
  Error : Inport
  BD : Inport  Port=2
  Add : Sum  Inputs=+++  OutDataTypeStr=single  RndMeth=Nearest
  Add1 : Sum  Inputs=-+  OutDataTypeStr=single  RndMeth=Nearest
  Add2 : Sum  OutDataTypeStr=single  RndMeth=Nearest
  Derivative : Subsystem  mask{Ts_=Ts_}
      mask prompts: Ts_ "Sampling Time"
      mask init:
      | Ts_=Ts_;
      mask Display: dpoly([1 -1],[0 Ts_],'z')
  Fillter : Subsystem
  Gain4 : Gain  Gain=0.1
  Gain5 : Gain  Gain=0.01
  Gain6 : Gain  Gain=0.01
  Gain7 : Gain  Gain=0.01
  I_over_guard : Subsystem
  Integrator : Subsystem  mask{Ts_=Ts_}
      mask prompts: Ts_ "Sampling Time"
      mask Display: dpoly([Ts_],[1 -1],'z')
  Product{,1..3} (4 alike) : Product  RndMeth=Zero
  Saturation : Saturate  UpperLimit=SaturationMax  LowerLimit=SaturationMin  LinearizeAsGain=off  OutDataTypeStr=single  RndMeth=Nearest
  Scope : Scope  NumInputPorts=3
      settings: YMin=-5~-5~-5  YMax=5~5~5  SaveName=ScopeData5
  Scope1 : Scope  NumInputPorts=2
      settings: YMin=-5~-5  YMax=5~5  SaveName=ScopeData6
  Selector1 : Selector  InputPortWidth=5  IndexOptions=Index vector (dialog)  Indices=1  OutputSizes=1
  Selector2 : Selector  InputPortWidth=5  IndexOptions=Index vector (dialog)  Indices=2  OutputSizes=1
  Selector3 : Selector  InputPortWidth=5  IndexOptions=Index vector (dialog)  Indices=3  OutputSizes=1
  Selector4 : Selector  InputPortWidth=5  IndexOptions=Index vector (dialog)  Indices=4  OutputSizes=1
  Selector5 : Selector  InputPortWidth=5  IndexOptions=Index vector (dialog)  Indices=5  OutputSizes=1
  Target_deg : Outport
  wires:
  Product/1 -> Add2/2
  Add1/1 -> Product/1
  Add2/1 -> Integrator/1(In)
  Product1/1 -> Add/1, Scope/1
  Integrator/1(Out) -> Add/2, Scope/2
  Add/1 -> Add1/1, Saturation/1
  Derivative/1(Out) -> I_over_guard/1(In1)
  Product2/1 -> Add2/1
  Product3/1 -> Scope1/1, Fillter/1(In)
  Saturation/1 -> Add1/2, Target_deg/1
  Selector1/1 -> Gain4/1
  Selector2/1 -> Gain5/1
  Selector3/1 -> Gain6/1
  Selector4/1 -> Gain7/1
  Gain4/1 -> [P]
  Gain5/1 -> [I]
  Gain6/1 -> [D]
  Gain7/1 -> [B]
  [B] -> Product/2
  [P] -> Product1/2
  [I] -> Product2/2
  [D] -> Product3/2
  BD/1 -> Selector2/1, Selector3/1, Selector4/1, Selector1/1, Selector5/1
  Error/1 -> Product1/1, Product2/1, Product3/1
  I_over_guard/1(Out1) -> Add/3, Scope/3, Scope1/2
  Fillter/1(Out) -> Derivative/1(In)
  Selector5/1 -> Fillter/2(In1)

== system et_robocon_dev_guy_arch_pi/Main Controller/normal_operation_modes.line_tracking_mode/line_tracking_mode.balanceControl/ForSimulation/Cal_PWM ==
  note: Calculate maximum of DC motor
      | voltatege from battery using an
      | experimental expression.
  note: Turn NXTway-GS by applying pwm offset
      | to left and right motor in the counter direction.
  pwm_turn : Inport
  err : Inport  Port=2
  battery : Inport  Port=3
  Cal_vol_max : Subsystem
  Gain : Gain  Gain=100  OutDataTypeStr=Inherit: Same as input  ParamDataTypeStr=Inherit: Same as input
  Product : Product  Inputs=*/  RndMeth=Simplest  OutDataTypeStr=Inherit: Same as first input
  Sum : Sum  Inputs=|++  OutDataTypeStr=Inherit: Same as first input
  Sum1 : Sum  Inputs=|+-  OutDataTypeStr=Inherit: Same as first input
  pwm_l_limiter : Saturate  UpperLimit=100  LowerLimit=-100
      settings: AttributesFormatString=max = %<UpperLimit>\nmin = %<LowerLimit>
  pwm_r_limiter : Saturate  UpperLimit=100  LowerLimit=-100
      settings: AttributesFormatString=max = %<UpperLimit>\nmin = %<LowerLimit>
  pwm_l : Outport
  pwm_r : Outport  Port=2
  wires:
  Sum/1 -> pwm_l_limiter/1
  pwm_turn/1 -> Sum/2, Sum1/2
  Gain/1 -> Sum1/1, Sum/1
  err/1 -> Product/1
  Product/1 -> Gain/1
  battery/1 -> Cal_vol_max/1(battery)
  Cal_vol_max/1(vol_max) -> Product/2
  Sum1/1 -> pwm_r_limiter/1
  pwm_r_limiter/1 -> pwm_r/1
  pwm_l_limiter/1 -> pwm_l/1

== system et_robocon_dev_guy_arch_pi/Main Controller/normal_operation_modes.line_tracking_mode/line_tracking_mode.balanceControl/ForSimulation/Cal_Reference ==
  note: Divide command values by
      | maximum of command input.
  note: Smooth velocity command
      | using Low Path Filter to
      | suppress rapid input change.
  cmd_forward : Inport
  cmd_turn : Inport  Port=2
  Constant1 : Constant  Value=cmd_max  VectorParams1D=off  OutDataTypeStr=single  SampleTime=-1
      settings: AttributesFormatString=DataType = %<OutDataTypeStr>
  Constant2 : Constant  Value=0  VectorParams1D=off  OutDataTypeStr=single  SampleTime=-1
      settings: AttributesFormatString=DataType = %<OutDataTypeStr>
  Constant3 : Constant  Value=0  VectorParams1D=off  OutDataTypeStr=single  SampleTime=-1
      settings: AttributesFormatString=DataType = %<OutDataTypeStr>
  Constant6 : Constant  Value=cmd_max  VectorParams1D=off  OutDataTypeStr=single  SampleTime=-1
      settings: AttributesFormatString=DataType = %<OutDataTypeStr>
  DiscreteIntegrator : Subsystem
  Divide : Product  Inputs=*/  RndMeth=Simplest  OutDataTypeStr=Inherit: Same as first input
  Divide1 : Product  Inputs=*/  RndMeth=Simplest  OutDataTypeStr=Inherit: Same as first input
  Gain1 : Gain  Gain=k_thetadot  OutDataTypeStr=Inherit: Same as input  ParamDataTypeStr=Inherit: Same as input
  Gain2 : Gain  Gain=k_phidot  OutDataTypeStr=Inherit: Same as input  ParamDataTypeStr=Inherit: Same as input
  LowPathFilter : Subsystem
  Mux : Mux
  pwm_turn : Outport
  theta_ref : Outport  Port=2
  x1_ref : Outport  Port=3
  wires:
  cmd_turn/1 -> Divide1/1
  Gain1/1 -> LowPathFilter/1(in)
  cmd_forward/1 -> Divide/1
  Divide/1 -> Gain1/1
  Gain2/1 -> pwm_turn/1  "pwm_turn"
  Constant1/1 -> Divide1/2
  Divide1/1 -> Gain2/1
  Mux/1 -> x1_ref/1
  DiscreteIntegrator/1(out) -> theta_ref/1, Mux/1  "theta_ref"
  Constant2/1 -> Mux/2  "psi_ref"
  Constant3/1 -> Mux/4  "psidot_ref"
  LowPathFilter/1(out) -> Mux/3, DiscreteIntegrator/1(in)  "thetadot_ref"
  Constant6/1 -> Divide/2

== system et_robocon_dev_guy_arch_pi/Main Controller/normal_operation_modes.line_tracking_mode/line_tracking_mode.balanceControl/ForSimulation/Cal_x1 ==
  note: Smooth measured velocity value using
      | Low Path Filter to reduce the noise
      | because it makes extra control input.
  note: Calculate gyro offset for removing gyro drift.
  gyro : Inport
  gyro_offset : Inport  Port=2
  theta_m_l : Inport  Port=3
  theta_m_r : Inport  Port=4
  DiscreteDerivative : Subsystem
  DiscreteIntegrator : Subsystem
  Gain : Gain  Gain=1/2  OutDataTypeStr=Inherit: Same as input  ParamDataTypeStr=Inherit: Same as input
  LowPathFilter : Subsystem
  Mux1 : Mux
  Sum1 : Sum  Inputs=++|  OutDataTypeStr=Inherit: Same as first input
  Sum2 : Sum  Inputs=|+-  OutDataTypeStr=Inherit: Same as first input
  Sum4 : Sum  Inputs=|++  OutDataTypeStr=Inherit: Same as first input
  Sum6 : Sum  Inputs=|++  OutDataTypeStr=Inherit: Same as first input
  deg2rad : Gain  Gain=deg2rad  OutDataTypeStr=Inherit: Same as input  ParamDataTypeStr=Inherit: Same as input
  deg2rad1 : Gain  Gain=deg2rad  OutDataTypeStr=Inherit: Same as input  ParamDataTypeStr=Inherit: Same as input
  deg2rad2 : Gain  Gain=deg2rad  OutDataTypeStr=Inherit: Same as input  ParamDataTypeStr=Inherit: Same as input
  theta : Outport
  x1 : Outport  Port=2
  wires:
  deg2rad1/1 -> Sum4/1
  Mux1/1 -> x1/1
  DiscreteIntegrator/1(out) -> Sum6/2, Sum4/2, Mux1/2  "psi"
  deg2rad/1 -> Sum6/1
  theta_m_l/1 -> deg2rad/1
  theta_m_r/1 -> deg2rad1/1
  DiscreteDerivative/1(out) -> Mux1/3  "thetadot"
  Sum6/1 -> Sum1/1  "theta_l"
  Sum4/1 -> Sum1/2  "theta_r"
  Sum1/1 -> Gain/1  "thata_m_sum"
  gyro/1 -> Sum2/1
  Sum2/1 -> deg2rad2/1
  deg2rad2/1 -> Mux1/4, DiscreteIntegrator/1(in)  "psidot"
  LowPathFilter/1(out) -> DiscreteDerivative/1(in)
  Gain/1 -> theta/1, Mux1/1, LowPathFilter/1(in)  "theta"
  gyro_offset/1 -> Sum2/2
  LowPathFilter/2(out1) -> DiscreteDerivative/2(in1)

== system et_robocon_dev_guy_arch_pi/Main Controller/normal_operation_modes.line_tracking_mode/line_tracking_mode.balanceControl/ForSimulation/DiscreteIntegrator ==
  in : Inport
  Gain : Gain  Gain=exec_period  OutDataTypeStr=Inherit: Same as input  ParamDataTypeStr=Inherit: Same as input
  Sum : Sum  Inputs=|++  OutDataTypeStr=Inherit: Same as first input
  Unit Delay : UnitDelay  SampleTime=-1  StateName=ud_psi  StateMustResolveToSignalObject=on
      settings: AttributesFormatString=Signal name = ud_psi
  out : Outport
  wires:
  Unit Delay/1 -> Sum/2, out/1
  Gain/1 -> Sum/1
  Sum/1 -> Unit Delay/1
  in/1 -> Gain/1

== system et_robocon_dev_guy_arch_pi/Main Controller/normal_operation_modes.line_tracking_mode/line_tracking_mode.balanceControl/Low Pass Filter/Store Offset ==
  x : Inport
  Enable : EnablePort
  x0 : Outport  InitialOutput=0
  wires:
  x/1 -> x0/1

== system et_robocon_dev_guy_arch_pi/State Estimation/Data Type Conversion Unit Conversion Tail Initialization/Low Pass Filter/Store Offset ==
  x : Inport
  Enable : EnablePort
  x0 : Outport  InitialOutput=0
  wires:
  x/1 -> x0/1

== system et_robocon_dev_guy_arch_pi/State Estimation/Data Type Conversion Unit Conversion Tail Initialization/tail processing/tail initialization ==
  tail : Inport
  Trigger : TriggerPort  PortDimensions=1
  tail_0 : Outport  InitialOutput=0
  wires:
  tail/1 -> tail_0/1

== system et_robocon_dev_guy_arch_pi/State Estimation/Gyro Processing/Compute psi/Very Low Pass Filter ==
  In1 : Inport
  Gain2 : Gain  Gain=0.004
  Gain3 : Gain  Gain=0.996
  Sum2 : Sum  Inputs=|++
  Unit Delay External IC : simulink/Additional Math & Discrete/Additional Discrete/Unit Delay External IC  tsamp=-1
  Out1 : Outport
  wires:
  Gain3/1 -> Sum2/2
  Sum2/1 -> Out1/1, Unit Delay External IC/1
  Gain2/1 -> Sum2/1
  Unit Delay External IC/1 -> Gain3/1
  In1/1 -> Gain2/1, Unit Delay External IC/2

== system et_robocon_dev_guy_arch_pi/State Estimation/StateEstimation/Process theta1/Enabled Subsystem ==
  x : Inport
  Enable : EnablePort
  x0 : Outport  InitialOutput=0
  wires:
  x/1 -> x0/1

== system et_robocon_dev_guy_arch_pi/State Estimation/StateEstimation/Process theta1/LPF and deriv ==
  theta : Inport
  Gain : Gain  Gain=1/0.004
  Low Pass Filter : DiscreteFilter  Numerator=[.2]  Denominator=[1 -0.8]
  Sum3 : Sum  Inputs=+-
  Unit Delay : UnitDelay  SampleTime=-1
  theta_dot : Outport
  wires:
  Unit Delay/1 -> Sum3/2
  Gain/1 -> Unit Delay/1, Sum3/1
  Sum3/1 -> theta_dot/1  "theta_dot"
  Low Pass Filter/1 -> Gain/1
  theta/1 -> Low Pass Filter/1

== system et_robocon_dev_guy_arch_pi/State Estimation/StateEstimation/Process theta1/LPF and deriv1 ==
  theta_dot : Inport
  Gain : Gain  Gain=1/0.004
  Low Pass Filter : DiscreteFilter  Numerator=[.2]  Denominator=[1 -0.8]
  Sum3 : Sum  Inputs=+-
  Unit Delay : UnitDelay  SampleTime=-1
  theta_dot_dot : Outport
  wires:
  theta_dot/1 -> Low Pass Filter/1
  Low Pass Filter/1 -> Gain/1
  Sum3/1 -> theta_dot_dot/1  "theta_dot_dot"
  Gain/1 -> Sum3/1, Unit Delay/1
  Unit Delay/1 -> Sum3/2

== system et_robocon_dev_guy_arch_pi/State Estimation/StateEstimation/Process theta1/Store x0 ==
  x : Inport
  Enable : EnablePort
  x0 : Outport  InitialOutput=0
  wires:
  x/1 -> x0/1

== system et_robocon_dev_guy_arch_pi/Main Controller/normal_operation_modes.line_tracking_after_seesaw/line_tracking_mode.Track.lineTracker/SwitchForFreeSteering/tmpController/Derivative ==
  In : Inport
  Constant2 : Constant  Value=Ts_  OutDataTypeStr=single  SampleTime=-1
  Difference : simulink/Discrete/Difference  ICPrevInput=0.0  InputProcessing=Inherited  OutMin=[]  OutMax=[]  OutDataTypeStr=single  OutputDataTypeScalingMode=single  OutDataType=sfix(16)  OutScaling=2^-10  RndMeth=Nearest  DoSatur=off
  Divide4 : Product  Inputs=*/  OutDataTypeStr=single  RndMeth=Nearest
  Out : Outport
  wires:
  Constant2/1 -> Divide4/2
  Divide4/1 -> Difference/1
  In/1 -> Divide4/1
  Difference/1 -> Out/1

== system et_robocon_dev_guy_arch_pi/Main Controller/normal_operation_modes.line_tracking_after_seesaw/line_tracking_mode.Track.lineTracker/SwitchForFreeSteering/tmpController/Fillter ==
  In : Inport
  In1 : Inport  Port=2
  Add : Sum  RndMeth=Nearest
  Add2 : Sum  Inputs=+-  OutDataTypeStr=single  RndMeth=Nearest
  Constant : Constant  Value=single(1-(0.0001/(0.1*Ts_)))  OutDataTypeStr=single  SampleTime=-1
  Constant1 : Constant  Value=single(0.0001/(0.1*Ts_))  OutDataTypeStr=single  SampleTime=-1
  Constant2 : Constant  Value=(0.1*Ts_)  OutDataTypeStr=single  SampleTime=-1
  Constant3 : Constant  OutDataTypeStr=single  SampleTime=-1
  Constant4 : Constant  Value=0.00001  OutDataTypeStr=single  SampleTime=-1
  Constant6 : Constant  Value=(0.1*Ts_)  OutDataTypeStr=single  SampleTime=-1
  Divide : Product  Inputs=*/
  Divide1 : Product  Inputs=*/
  Manual Switch1 : ManualSwitch  CurrentSetting=0
  Manual Switch3 : ManualSwitch  CurrentSetting=0
  Product : Product  OutDataTypeStr=single  RndMeth=Nearest
  Product1 : Product  OutDataTypeStr=single  RndMeth=Nearest
  Product3 : Product  OutDataTypeStr=single  RndMeth=Nearest
  Unit Delay : UnitDelay  SampleTime=-1
  Unit Delay1 : UnitDelay  SampleTime=-1
  Out : Outport
  wires:
  In/1 -> Unit Delay1/1
  Unit Delay1/1 -> Product1/1
  Product1/1 -> Add/1
  Unit Delay/1 -> Product/2
  Add/1 -> Out/1, Unit Delay/1
  Product/1 -> Add/2
  Constant6/1 -> Divide/2
  Constant2/1 -> Divide1/2
  Divide1/1 -> Add2/2
  In1/1 -> Product3/1
  Product3/1 -> Divide1/1, Divide/1
  Constant4/1 -> Product3/2
  Constant3/1 -> Add2/1
  Manual Switch1/1 -> Product1/2
  Constant1/1 -> Manual Switch1/1
  Divide/1 -> Manual Switch1/2
  Manual Switch3/1 -> Product/1
  Constant/1 -> Manual Switch3/1
  Add2/1 -> Manual Switch3/2

== system et_robocon_dev_guy_arch_pi/Main Controller/normal_operation_modes.line_tracking_after_seesaw/line_tracking_mode.Track.lineTracker/SwitchForFreeSteering/tmpController/I_over_guard ==
  In1 : Inport
  Compare To Constant1 : simulink/Logic and Bit Operations/Compare To Constant  relop===  const=1  OutDataTypeStr=uint8
  Constant2 : Constant  Value=0  OutDataTypeStr=uint8  SampleTime=-1
  Constant4 : Constant  Value=0  OutDataTypeStr=uint8  SampleTime=-1
  Memory1 : Memory  X0=1  InheritSampleTime=on
  Switch : Switch  Threshold=1
  Out1 : Outport
  wires:
  Memory1/1 -> Compare To Constant1/1
  Constant2/1 -> Memory1/1
  Constant4/1 -> Switch/1
  Compare To Constant1/1 -> Switch/2
  Switch/1 -> Out1/1
  In1/1 -> Switch/3

== system et_robocon_dev_guy_arch_pi/Main Controller/normal_operation_modes.line_tracking_after_seesaw/line_tracking_mode.Track.lineTracker/SwitchForFreeSteering/tmpController/Integrator ==
  In : Inport
  Constant2 : Constant  Value=Ts_  OutDataTypeStr=single  SampleTime=-1
  Integrator : DiscreteTransferFcn  Denominator=[1 -1]  RndMeth=Nearest
  Product1 : Product  OutDataTypeStr=single  RndMeth=Nearest
  Out : Outport
  wires:
  Constant2/1 -> Product1/2
  Product1/1 -> Integrator/1
  In/1 -> Product1/1
  Integrator/1 -> Out/1

== system et_robocon_dev_guy_arch_pi/Main Controller/normal_operation_modes.line_tracking_after_seesaw/line_tracking_mode.balanceControl/ForSimulation/Cal_PWM/Cal_vol_max ==
  battery : Inport
  Constant : Constant  Value=battery_offset  OutDataTypeStr=single  SampleTime=-1
      settings: AttributesFormatString=DataType = %<OutDataTypeStr>
  Gain3 : Gain  Gain=battery_gain  OutDataTypeStr=Inherit: Same as input  ParamDataTypeStr=Inherit: Same as input
  Sum2 : Sum  Inputs=|+-  OutDataTypeStr=Inherit: Same as first input
  vol_max : Outport
  wires:
  Constant/1 -> Sum2/2
  Sum2/1 -> vol_max/1  "base_pwm"
  Gain3/1 -> Sum2/1
  battery/1 -> Gain3/1
